simulink model "lorenz_model"  (R2018a)
settings: Solver=FixedStepAuto  StartTime=0.0  StopTime=inf  RelTol=1e-3  EnableMultiTasking=on
undefined symbols (not defined in the file): DiscIntNeverNeededParam
libraries: simulink x7, simulink_extras x1
settings Model: Creator=labuser  LastModifiedBy=labuser
settings SolverCC: PositivePriorityOrder=on  AutoInsertRateTranBlk=on
settings OptimizationCC: BlockReduction=off  ConditionallyExecuteInputs=off  DefaultParameterBehavior=Inlined  EnhancedBackFolding=on  PassReuseOutputArgsThreshold=0  MaxStackSize=64  OptimizeBlockOrder=speed  DifferentSizesBufferReuse=on  OptimizationCustomize=off
settings DebuggingCC: AlgebraicLoopMsg=error  ParameterTunabilityLossMsg=error
settings HardwareCC: ProdBitPerPointer=32  ProdBitPerSizeT=32  ProdBitPerPtrDiffT=32  ProdLargestAtomicFloat=None  ProdIntDivRoundTo=Undefined  ProdEndianess=Unspecified  ProdWordSize=32  ProdHWDeviceType=ASIC/FPGA->ASIC/FPGA  TargetBitPerPointer=64  TargetBitPerSizeT=64  TargetBitPerPtrDiffT=64  TargetLongLongMode=on  TargetIntDivRoundTo=Zero  TargetEndianess=LittleEndian  TargetWordSize=64  TargetHWDeviceType=Custom Processor->MATLAB Host Computer  ProdEqTarget=off
settings SFSimCC: MATLABDynamicMemAlloc=off
settings RTWCC: Description=Generic Real-Time Target  GenerateReport=on  Toolchain=ARM Development Studio Altera Edition (DS-5 AE)  LaunchReport=on
settings CodeAppCC: ForceParamTrailComments=on  OperatorAnnotations=on
settings GRTTargetCC: TargetLangStandard=C89/C90 (ANSI)

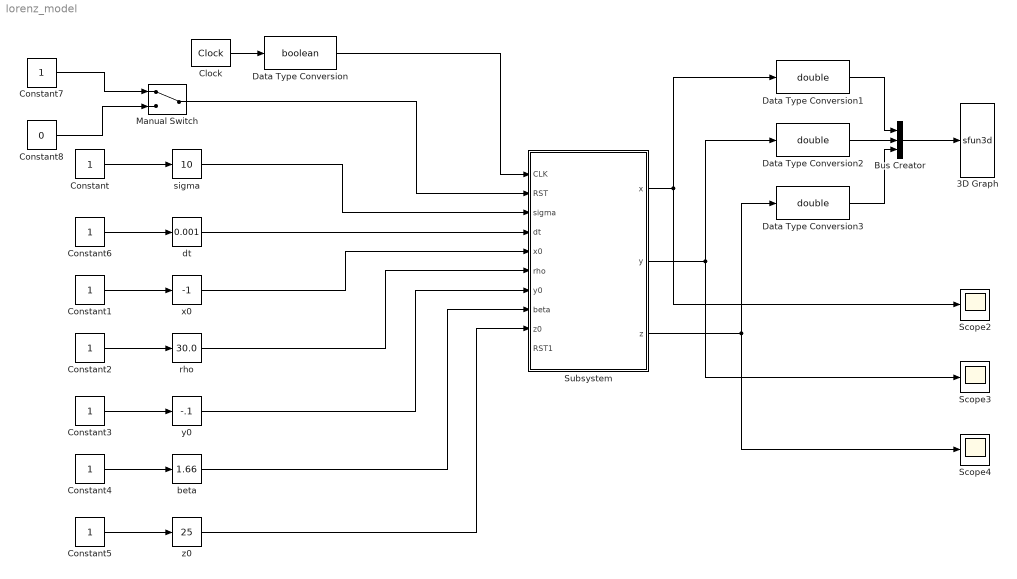
== system lorenz_model ==
  3D Graph : S-Function  LoadFcn=if exist('sfun3d','file'), sfun3d([],[],[],'LoadBlock'); end  FunctionName=sfun3d  Parameters=ax,T,np,cp,gd,ls,mk,mx,hd,tb  SFunctionDeploymentMode=off  EnableBusSupport=off  mask(3D Graph){np=1, ax=[-30 30 -30 30 0 50], mx=2000, T=0.01, cp=[370 -234 -207], gd=on, hd=on, tb=off, ls=-, mk=none}
      mask prompts: np "Number of moving points (lines)"; ax "Range: [xmin xmax  ymin ymax zmin zmax]"; mx "Max number of points in each line"; T "Sampling Time"; cp "Camera position (use [0 0 1] for 2D XY view)"; gd "Grid (on|off)"; hd "HeadMarkers (on|off)"; tb "Toolbar (on|off)"; ls "LineStyle"; mk "LineMarker"
      mask help:
      | This block plots the position of several points in the XYZ space. The input contains the coordinates of all the points (x1,y1,z1,x2,y2,z2,...).
      | The number of moving points (lines), the XYZ ranges, sampling time, camera position, and grid (among other things) can be set as mask parameters.
      settings: CopyFcn=if exist('sfun3d','file'), sfun3d([],[],[],'CopyBlock'); end  DeleteFcn=if exist('sfun3d','file'), sfun3d([],[],[],'DeleteBlock'); end  NameChangeFcn=if exist('sfun3d','file'), sfun3d([],[],[],'NameChange'); end
      mask Help:
      | This block plots the position of several points in the XYZ space. The input contains the coordinates of all the points (x1,y1,z1,x2,y2,z2,...).
      | The number of moving points (lines), the XYZ ranges, sampling time, camera position, and grid (among other things) can be set as mask parameters.
      mask TypeOptions ls: - | -- | : | -. | none
      mask TypeOptions mk: none | . | + | o | * | x | square | diamond | v | ^ | > | < | pentagram | hexagram
      mask Display: plot([.05 .95 .95 .05 .05],[.45 .45 .95 .95 .45], 0.5+cos(0:0.1:2*pi)*0.3,0.7+sin(0:0.1:2*pi)*0.2)
  Bus Creator : BusCreator  Inputs=3
  Clock : simulink_extras/Flip Flops/Clock  period=0.001
  Constant{,1..6} (7 alike) : Constant  OutDataTypeStr=fixdt(1,27,20)  SampleTime=-1
  Constant7 : Constant  OutDataTypeStr=boolean  SampleTime=-1
  Constant8 : Constant  Value=0  OutDataTypeStr=boolean  SampleTime=-1
  Data Type Conversion : DataTypeConversion  OutDataTypeStr=boolean
  Data Type Conversion1 : DataTypeConversion  OutDataTypeStr=double
  Data Type Conversion2 : DataTypeConversion  OutDataTypeStr=double
  Data Type Conversion3 : DataTypeConversion  OutDataTypeStr=double
  Manual Switch : ManualSwitch
  Scope2 : Scope
  Scope3 : Scope
  Scope4 : Scope
  Subsystem : Subsystem  TreatAsAtomicUnit=on
  beta : simulink/Math Operations/Slider Gain  gain=1.66  low=0  high=5
  dt : simulink/Math Operations/Slider Gain  gain=0.001  low=0  high=100
  rho : simulink/Math Operations/Slider Gain  gain=30.0  low=0  high=50
  sigma : simulink/Math Operations/Slider Gain  gain=10  low=-20  high=20
  x0 : simulink/Math Operations/Slider Gain  gain=-1  low=-2  high=2
  y0 : simulink/Math Operations/Slider Gain  gain=-.1  low=-1  high=1
  z0 : simulink/Math Operations/Slider Gain  gain=25  low=0  high=50
  wires:
  Constant7/1 -> Manual Switch/1
  Constant8/1 -> Manual Switch/2
  Manual Switch/1 -> Subsystem/2(RST)
  Clock/1 -> Data Type Conversion/1
  Data Type Conversion/1 -> Subsystem/1(CLK)
  Bus Creator/1 -> 3D Graph/1
  Data Type Conversion1/1 -> Bus Creator/1
  Data Type Conversion2/1 -> Bus Creator/2
  Data Type Conversion3/1 -> Bus Creator/3
  sigma/1 -> Subsystem/3(sigma)
  Constant1/1 -> x0/1
  Constant2/1 -> rho/1
  Constant5/1 -> z0/1
  Constant3/1 -> y0/1
  Constant6/1 -> dt/1
  Constant4/1 -> beta/1
  Constant/1 -> sigma/1
  dt/1 -> Subsystem/4(dt)
  x0/1 -> Subsystem/5(x0)
  rho/1 -> Subsystem/6(rho)
  y0/1 -> Subsystem/7(y0)
  z0/1 -> Subsystem/9(z0)
  beta/1 -> Subsystem/8(beta)
  Subsystem/1(x) -> Data Type Conversion1/1, Scope2/1
  Subsystem/3(z) -> Scope4/1, Data Type Conversion3/1
  Subsystem/2(y) -> Scope3/1, Data Type Conversion2/1

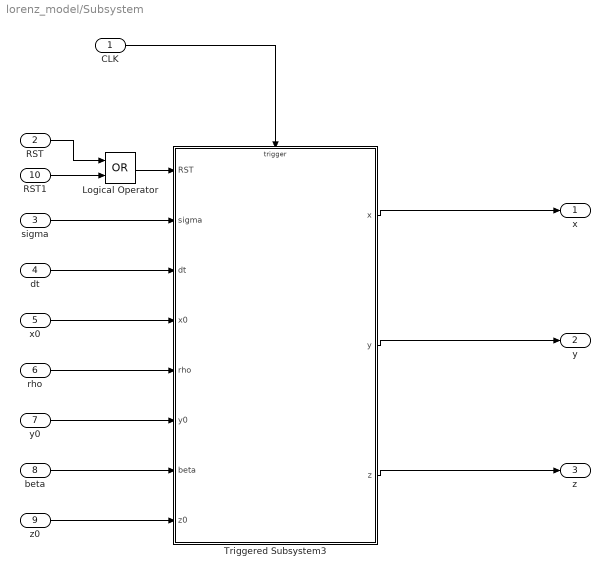
== system lorenz_model/Subsystem ==
  CLK : Inport  OutDataTypeStr=boolean
  RST : Inport  Port=2  OutDataTypeStr=boolean
  sigma : Inport  Port=3  OutDataTypeStr=fixdt(1,27,20)
  dt : Inport  Port=4  OutDataTypeStr=fixdt(1,27,20)
  x0 : Inport  Port=5  OutDataTypeStr=fixdt(1,27,20)
  rho : Inport  Port=6  OutDataTypeStr=fixdt(1,27,20)
  y0 : Inport  Port=7  OutDataTypeStr=fixdt(1,27,20)
  beta : Inport  Port=8  OutDataTypeStr=fixdt(1,27,20)
  z0 : Inport  Port=9  OutDataTypeStr=fixdt(1,27,20)
  RST1 : Inport  Port=10  OutDataTypeStr=boolean
  Logical Operator : Logic  Operator=OR  AllPortsSameDT=off  OutDataTypeStr=boolean
  Triggered Subsystem3 : Subsystem  TreatAsAtomicUnit=on
  x : Outport  OutDataTypeStr=fixdt(1,27,20)
  y : Outport  Port=2  OutDataTypeStr=fixdt(1,27,20)
  z : Outport  Port=3  OutDataTypeStr=fixdt(1,27,20)
  wires:
  Triggered Subsystem3/3(z) -> z/1
  Triggered Subsystem3/2(y) -> y/1
  Triggered Subsystem3/1(x) -> x/1
  CLK/1 -> Triggered Subsystem3/Trigger
  RST/1 -> Logical Operator/1
  sigma/1 -> Triggered Subsystem3/2(sigma)
  dt/1 -> Triggered Subsystem3/3(dt)
  x0/1 -> Triggered Subsystem3/4(x0)
  rho/1 -> Triggered Subsystem3/5(rho)
  y0/1 -> Triggered Subsystem3/6(y0)
  beta/1 -> Triggered Subsystem3/7(beta)
  z0/1 -> Triggered Subsystem3/8(z0)
  Logical Operator/1 -> Triggered Subsystem3/1(RST)
  RST1/1 -> Logical Operator/2

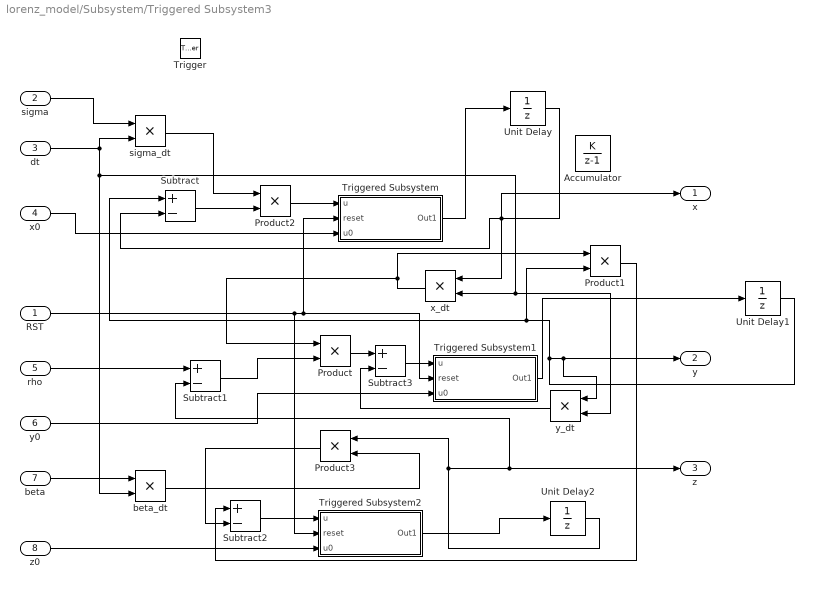
== system lorenz_model/Subsystem/Triggered Subsystem3 ==
  RST : Inport  OutDataTypeStr=boolean
  sigma : Inport  Port=2  OutDataTypeStr=fixdt(1,27,20)
  dt : Inport  Port=3  OutDataTypeStr=fixdt(1,27,20)
  x0 : Inport  Port=4  OutDataTypeStr=fixdt(1,27,20)
  rho : Inport  Port=5  OutDataTypeStr=fixdt(1,27,20)
  y0 : Inport  Port=6  OutDataTypeStr=fixdt(1,27,20)
  beta : Inport  Port=7  OutDataTypeStr=fixdt(1,27,20)
  z0 : Inport  Port=8  OutDataTypeStr=fixdt(1,27,20)
  Trigger : TriggerPort  VariantControl=Variant
  Accumulator : DiscreteIntegrator  IntegratorMethod=Accumulation: Forward Euler  SampleTime=-1  ICPrevOutput=DiscIntNeverNeededParam  ICPrevScaledInput=DiscIntNeverNeededParam
  Product{,1..3} (4 alike) : Product  OutDataTypeStr=fixdt(1,27,20)
  Subtract{,1..3} (4 alike) : Sum  Inputs=+-  AccumDataTypeStr=fixdt(1,27,20)
  Triggered Subsystem : Subsystem  TreatAsAtomicUnit=on
  Triggered Subsystem1 : Subsystem  TreatAsAtomicUnit=on
  Triggered Subsystem2 : Subsystem  TreatAsAtomicUnit=on
  Unit Delay : UnitDelay  SampleTime=-1
  Unit Delay1 : UnitDelay  SampleTime=-1
  Unit Delay2 : UnitDelay  SampleTime=-1
  beta_dt : Product  OutDataTypeStr=fixdt(1,27,20)
  sigma_dt : Product  OutDataTypeStr=fixdt(1,27,20)
  x_dt : Product  OutDataTypeStr=fixdt(1,27,20)
  y_dt : Product  OutDataTypeStr=fixdt(1,27,20)
  x : Outport  OutDataTypeStr=fixdt(1,27,20)  InitialOutput=0
  y : Outport  Port=2  OutDataTypeStr=fixdt(1,27,20)  InitialOutput=0
  z : Outport  Port=3  OutDataTypeStr=fixdt(1,27,20)  InitialOutput=0
  wires:
  z0/1 -> Triggered Subsystem2/3(u0)
  Subtract3/1 -> Triggered Subsystem1/1(u)
  Unit Delay1/1 -> Subtract/1, Product1/2, y_dt/1, y/1
  Subtract2/1 -> Triggered Subsystem2/1(u)
  Product/1 -> Subtract3/1
  beta_dt/1 -> Product3/2
  Product3/1 -> Subtract2/2
  x_dt/1 -> Product1/1, Product/1
  y_dt/1 -> Subtract3/2
  RST/1 -> Triggered Subsystem2/2(reset), Triggered Subsystem1/2(reset), Triggered Subsystem/2(reset)
  beta/1 -> beta_dt/1
  Product1/1 -> Subtract2/1
  x0/1 -> Triggered Subsystem/3(u0)
  Unit Delay2/1 -> Product3/1, Subtract1/2, z/1
  y0/1 -> Triggered Subsystem1/3(u0)
  Subtract/1 -> Product2/2
  sigma/1 -> sigma_dt/1
  sigma_dt/1 -> Product2/1
  Subtract1/1 -> Product/2
  dt/1 -> sigma_dt/2, beta_dt/2, y_dt/2, x_dt/2
  Product2/1 -> Triggered Subsystem/1(u)
  rho/1 -> Subtract1/1
  Unit Delay/1 -> Subtract/2, x/1, x_dt/1
  Triggered Subsystem/1(Out1) -> Unit Delay/1
  Triggered Subsystem1/1(Out1) -> Unit Delay1/1
  Triggered Subsystem2/1(Out1) -> Unit Delay2/1

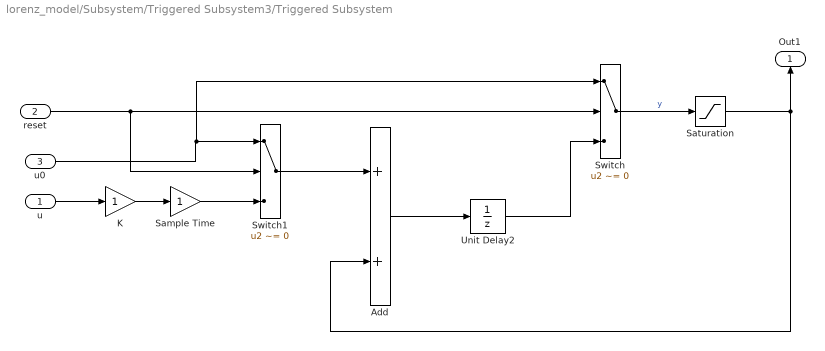
== system lorenz_model/Subsystem/Triggered Subsystem3/Triggered Subsystem ==
  u : Inport
  reset : Inport  Port=2
  u0 : Inport  Port=3
  Add : Sum
  K : Gain  OutDataTypeStr=Inherit: Same as input
  Sample Time : Gain  OutDataTypeStr=Inherit: Same as input
  Saturation : Saturate  UpperLimit=63  LowerLimit=-63
  Switch : Switch  Criteria=u2 ~= 0  OutDataTypeStr=Inherit: Inherit via back propagation
  Switch1 : Switch  Criteria=u2 ~= 0  OutDataTypeStr=Inherit: Inherit via back propagation
  Unit Delay2 : UnitDelay  SampleTime=-1
  Out1 : Outport
  wires:
  u/1 -> K/1
  u0/1 -> Switch/1, Switch1/1
  Switch1/1 -> Add/1
  Sample Time/1 -> Switch1/3
  Unit Delay2/1 -> Switch/3
  K/1 -> Sample Time/1
  Saturation/1 -> Out1/1, Add/2
  reset/1 -> Switch/2, Switch1/2
  Switch/1 -> Saturation/1  "y"
  Add/1 -> Unit Delay2/1

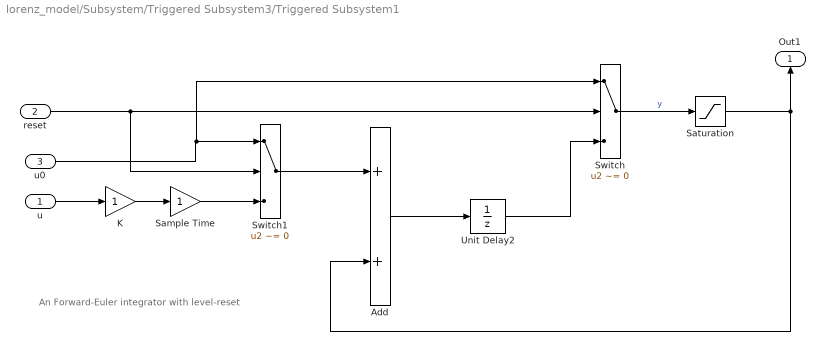
== system lorenz_model/Subsystem/Triggered Subsystem3/Triggered Subsystem1 ==
  note: An Forward-Euler integrator with level-reset
  u : Inport
  reset : Inport  Port=2
  u0 : Inport  Port=3
  Add : Sum
  K : Gain  OutDataTypeStr=Inherit: Same as input
  Sample Time : Gain  OutDataTypeStr=Inherit: Same as input
  Saturation : Saturate  UpperLimit=63  LowerLimit=-63
  Switch : Switch  Criteria=u2 ~= 0  OutDataTypeStr=Inherit: Inherit via back propagation
  Switch1 : Switch  Criteria=u2 ~= 0  OutDataTypeStr=Inherit: Inherit via back propagation
  Unit Delay2 : UnitDelay  SampleTime=-1
  Out1 : Outport
  wires:
  u/1 -> K/1
  u0/1 -> Switch/1, Switch1/1
  Switch1/1 -> Add/1
  Sample Time/1 -> Switch1/3
  Unit Delay2/1 -> Switch/3
  K/1 -> Sample Time/1
  Saturation/1 -> Out1/1, Add/2
  reset/1 -> Switch/2, Switch1/2
  Switch/1 -> Saturation/1  "y"
  Add/1 -> Unit Delay2/1

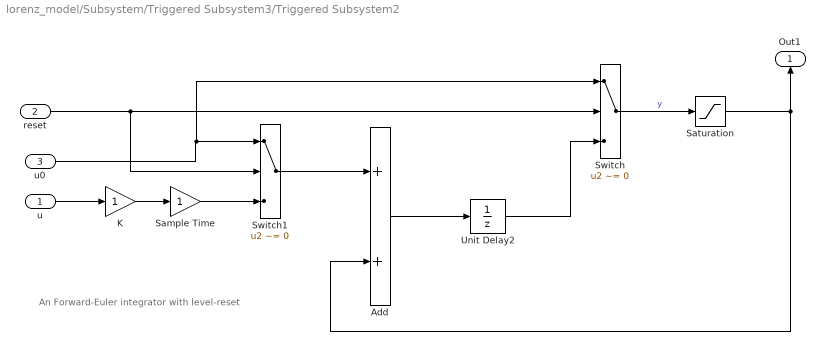
== system lorenz_model/Subsystem/Triggered Subsystem3/Triggered Subsystem2 ==
  note: An Forward-Euler integrator with level-reset
  u : Inport
  reset : Inport  Port=2
  u0 : Inport  Port=3
  Add : Sum
  K : Gain  OutDataTypeStr=Inherit: Same as input
  Sample Time : Gain  OutDataTypeStr=Inherit: Same as input
  Saturation : Saturate  UpperLimit=63  LowerLimit=-63
  Switch : Switch  Criteria=u2 ~= 0  OutDataTypeStr=Inherit: Inherit via back propagation
  Switch1 : Switch  Criteria=u2 ~= 0  OutDataTypeStr=Inherit: Inherit via back propagation
  Unit Delay2 : UnitDelay  SampleTime=-1
  Out1 : Outport
  wires:
  u/1 -> K/1
  u0/1 -> Switch/1, Switch1/1
  Switch1/1 -> Add/1
  Sample Time/1 -> Switch1/3
  Unit Delay2/1 -> Switch/3
  K/1 -> Sample Time/1
  Saturation/1 -> Out1/1, Add/2
  reset/1 -> Switch/2, Switch1/2
  Switch/1 -> Saturation/1  "y"
  Add/1 -> Unit Delay2/1
